simulink model "AircraftControlSystem 3"  (R2024b)
settings: Solver=VariableStepAuto  StartTime=0.0  StopTime=3  RelTol=1e-3
values from neighbouring files (symbols this model uses):
  A_at_eq = double(A_at_eq)    [AC_Model_Jacobian 3.m]
  B_at_eq = double(B_at_eq)    [AC_Model_Jacobian 3.m]
  C_tf = eye(12)    [AC_Model_Jacobian 3.m]
  D_tf = zeros(12, 4)    [AC_Model_Jacobian 3.m]
  Kd = -0.001*aero0    [AC_Model_Jacobian 3.m]
  Ki = 0.1*aero0    [AC_Model_Jacobian 3.m]
  Kp = 1*aero0    [AC_Model_Jacobian 3.m]
  u_cruise = 139    [AC_Model_Jacobian 3.m]
  X_ic = [0; 0; z_cruise; 0; 0; 0; u_cruise; 0; 0; 0; 0; 0]    [AC_Model_Jacobian 3.m]
libraries: simulink x1
settings Model: Creator=Hammad  LastModifiedBy=phill
settings DebuggingCC: UnconnectedInputMsg=warning  UnconnectedOutputMsg=warning  UnconnectedLineMsg=warning
settings ModelReferenceCC: EnableRefExpFcnMdlSchedulingChecks=on
settings RTWCC: GPUComputeCapability=3.5  DLArmComputeVersion=19.05

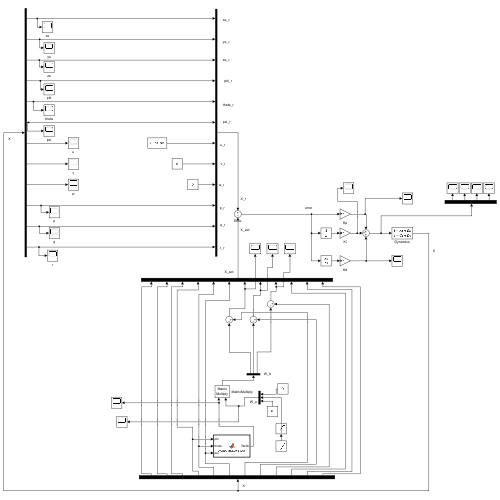
[thumbnail: Simulink's stored preview of the top-level diagram]
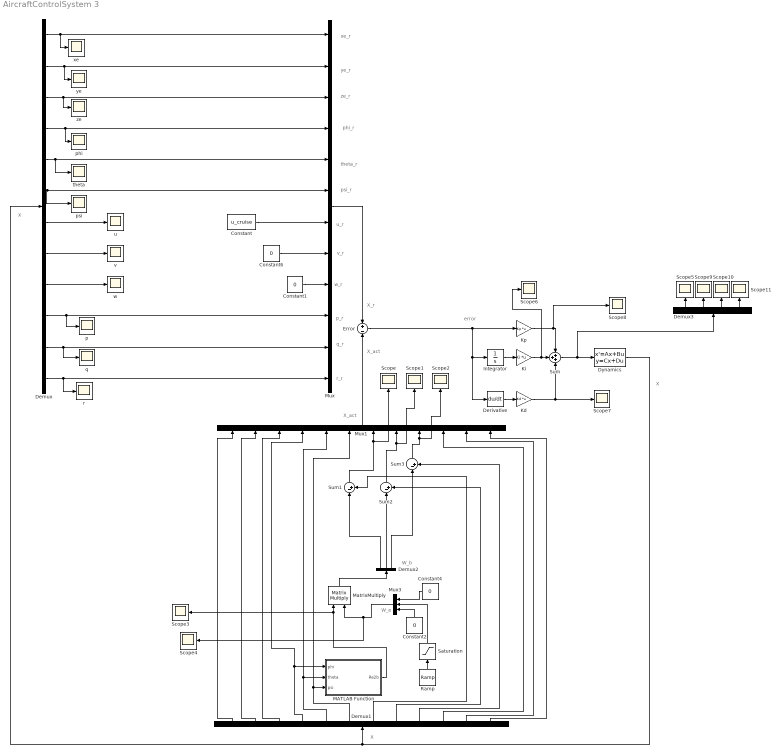
== system AircraftControlSystem 3 ==
  note: X
  note: error
  note: X_act
  note: X_r
  note: X
  note: W_b
  note: W_e
  note: xe_r
  note: ye_r
  note: ze_r
  note: psi_r
  note: theta_r
  note: phi_r
  note: w_r
  note: v_r
  note: u_r
  note: r_r
  note: q_r
  note: p_r
  note: X
  note: X_act
  Constant : Constant  Value=u_cruise
  Constant{1..2,4,6} (4 alike) : Constant  Value=0
  Demux : Demux  Outputs=12
  Demux1 : Demux  Outputs=12
  Demux2 : Demux  Outputs=3
  Demux3 : Demux
  Derivative : Derivative
  Dynamics : StateSpace  A=A_at_eq  B=B_at_eq  C=C_tf  D=D_tf  InitialCondition=X_ic
  Error : Sum  Inputs=+-
  Integrator : Integrator
  Kd : Gain  Gain=Kd  Multiplication=Matrix(K*u)
  Ki : Gain  Gain=Ki  Multiplication=Matrix(K*u)
  Kp : Gain  Gain=Kp  Multiplication=Matrix(K*u)
  MATLAB Function : MATLAB Function  TreatAsAtomicUnit=on
  MatrixMultiply : Product  Multiplication=Matrix(*)
  Mux : Mux  Inputs=12
  Mux1 : Mux  Inputs=12
  Mux3 : Mux  Inputs=3
  Ramp : simulink/Sources/Ramp  slope=1  start=1  InitialOutput=0
  Saturation : Saturate  UpperLimit=5  LowerLimit=0
  Scope{,1..11} (12 alike) : Scope
  Sum : Sum  Inputs=+++
  Sum1 : Sum  Inputs=|-+
  Sum2 : Sum  Inputs=|-+
  Sum3 : Sum  Inputs=|-+
  p : Scope
  phi : Scope
  psi : Scope
  q : Scope
  r : Scope
  theta : Scope
  u : Scope
  v : Scope
  w : Scope
  xe : Scope
  ye : Scope
  ze : Scope
  wires:
  Mux/1 -> Error/1
  Dynamics/1 -> Demux1/1, Demux/1
  Demux/1 -> Mux/1, xe/1
  Demux/2 -> Mux/2, ye/1
  Demux/4 -> Mux/4, phi/1
  Demux/5 -> theta/1, Mux/5
  Demux/6 -> Mux/6, psi/1
  Demux/12 -> Mux/12, r/1
  Demux/9 -> w/1
  Constant6/1 -> Mux/8
  Demux/8 -> v/1
  Demux/10 -> Mux/10, p/1
  Demux/11 -> Mux/11, q/1
  Derivative/1 -> Kd/1
  Integrator/1 -> Ki/1
  Kp/1 -> Scope8/1, Sum/1
  Ki/1 -> Scope6/1, Sum/2
  Kd/1 -> Sum/3, Scope7/1
  Demux/3 -> ze/1, Mux/3
  Demux/7 -> u/1
  Error/1 -> Kp/1, Derivative/1, Integrator/1
  Constant1/1 -> Mux/9
  Constant/1 -> Mux/7
  Demux1/1 -> Mux1/1
  Demux1/2 -> Mux1/2
  Demux1/3 -> Mux1/3
  Demux1/12 -> Mux1/12
  Demux1/11 -> Mux1/11
  Demux1/10 -> Mux1/10
  Sum3/1 -> Scope2/1, Mux1/9
  Sum2/1 -> Scope1/1, Mux1/8
  Mux1/1 -> Error/2
  Demux1/5 -> Mux1/5, MATLAB Function/2(theta)
  Demux1/4 -> Mux1/4, MATLAB Function/1(phi)
  Demux1/6 -> Mux1/6, MATLAB Function/3(psi)
  Constant4/1 -> Mux3/1
  Constant2/1 -> Mux3/3
  Mux3/1 -> Scope4/1, MatrixMultiply/2
  MATLAB Function/1(Re2b) -> Scope3/1, MatrixMultiply/1
  MatrixMultiply/1 -> Demux2/1
  Demux1/7 -> Sum1/2
  Demux1/8 -> Sum2/2
  Demux1/9 -> Sum3/2
  Demux2/1 -> Sum1/1
  Demux2/2 -> Sum2/1
  Demux2/3 -> Sum3/1
  Sum1/1 -> Mux1/7, Scope/1
  Ramp/1 -> Saturation/1
  Saturation/1 -> Mux3/2
  Demux3/3 -> Scope10/1
  Sum/1 -> Demux3/1, Dynamics/1
  Demux3/1 -> Scope5/1
  Demux3/2 -> Scope9/1
  Demux3/4 -> Scope11/1

== matlab function AircraftControlSystem 3/MATLAB Function ==
  data: phi input; Re2b output; theta input; psi input
function Re2b = computeRotation(phi, theta, psi)
    cphi = cos(phi);
    sphi = sin(phi);
    ctheta = cos(theta);
    stheta = sin(theta);
    cpsi = cos(psi);
    spsi = sin(psi);

    Re2b = [cpsi*ctheta, cpsi*stheta*sphi - spsi*cphi, cpsi*stheta*cphi + spsi*sphi;
         spsi*ctheta, spsi*stheta*sphi + cpsi*cphi, spsi*stheta*cphi - cpsi*sphi;
         -stheta,      ctheta*sphi,                 ctheta*cphi];
end
